simulink model "NoC_4x4x3"  (R2015a)
settings: Solver=ode45  StartTime=0.0  StopTime=10.0  RelTol=1e-3
undefined symbols (not defined in the file or in its folder): des, SELECT
undefined symbols (not defined in the file): MAX, MIN, T
libraries: simulink x48
(part 11 of 12)

== system NoC_4x4x3/LayerDown/Sitch3DXYZ/RouteXYZ/Attribute Function ==
  MATLAB Function : MATLAB Function  TreatAsAtomicUnit=on
  __DMLF__EDE2FCE__ : EntityDepartureFunctionCallGenerator  TimingFunctionCallF1=Before entity departure  IsInsideAFB=on
  __DMLF__GA__ : GetAttribute  AttributeName=DST_X|DST_Y|DST_Z|IME_X|IME_Y|IME_Z  AttributeMissing=Error|Error|Error|Error|Error|Error  AttributeDefaultValue=1|1|1|1|1|1  AttributeTreatAsVector=1|1|1|1|1|1  AttributeSendTiming=Before entity departure|Before entity departure|Before entity departure|Before entity departure|Before entity departure|Before entity departure  EvaluatedDefaultAttributeValue={ [];[];[];[];[];[]}  IsInsideAFB=on
      settings: OutputPortMap=o1,o2,o3,o4,o5,o6
  __DMLF__SA__ : SetAttribute  AttributeName=RT  AttributeFrom=Signal port  EvaluatedAttributeValue={ []}  IsInsideAFB=on
  IN : PMIOPort  Port=1  Side=Left
  OUT : PMIOPort  Port=2  Side=Right
  wires:
  __DMLF__EDE2FCE__/1 -> MATLAB Function/Trigger
  __DMLF__GA__/1 -> MATLAB Function/1(DST_X)
  __DMLF__GA__/2 -> MATLAB Function/2(DST_Y)
  __DMLF__GA__/3 -> MATLAB Function/3(DST_Z)
  __DMLF__GA__/4 -> MATLAB Function/4(IME_X)
  __DMLF__GA__/5 -> MATLAB Function/5(IME_Y)
  __DMLF__GA__/6 -> MATLAB Function/6(IME_Z)
  MATLAB Function/1(out_RT) -> __DMLF__SA__/1
  connections:
  __DMLF__SA__/RConn1 -- OUT/RConn1
  IN/RConn1 -- __DMLF__GA__/LConn1
  __DMLF__GA__/RConn1 -- __DMLF__EDE2FCE__/LConn1
  __DMLF__SA__/LConn1 -- __DMLF__EDE2FCE__/RConn1

== system NoC_4x4x3/LayerDown/Sitch3DXYZ1/RouteXYZ/Attribute Function ==
  MATLAB Function : MATLAB Function  TreatAsAtomicUnit=on
  __DMLF__EDE2FCE__ : EntityDepartureFunctionCallGenerator  TimingFunctionCallF1=Before entity departure  IsInsideAFB=on
  __DMLF__GA__ : GetAttribute  AttributeName=DST_X|DST_Y|DST_Z|IME_X|IME_Y|IME_Z  AttributeMissing=Error|Error|Error|Error|Error|Error  AttributeDefaultValue=1|1|1|1|1|1  AttributeTreatAsVector=1|1|1|1|1|1  AttributeSendTiming=Before entity departure|Before entity departure|Before entity departure|Before entity departure|Before entity departure|Before entity departure  EvaluatedDefaultAttributeValue={ [];[];[];[];[];[]}  IsInsideAFB=on
      settings: OutputPortMap=o1,o2,o3,o4,o5,o6
  __DMLF__SA__ : SetAttribute  AttributeName=RT  AttributeFrom=Signal port  EvaluatedAttributeValue={ []}  IsInsideAFB=on
  IN : PMIOPort  Port=1  Side=Left
  OUT : PMIOPort  Port=2  Side=Right
  wires:
  __DMLF__EDE2FCE__/1 -> MATLAB Function/Trigger
  __DMLF__GA__/1 -> MATLAB Function/1(DST_X)
  __DMLF__GA__/2 -> MATLAB Function/2(DST_Y)
  __DMLF__GA__/3 -> MATLAB Function/3(DST_Z)
  __DMLF__GA__/4 -> MATLAB Function/4(IME_X)
  __DMLF__GA__/5 -> MATLAB Function/5(IME_Y)
  __DMLF__GA__/6 -> MATLAB Function/6(IME_Z)
  MATLAB Function/1(out_RT) -> __DMLF__SA__/1
  connections:
  __DMLF__SA__/LConn1 -- __DMLF__EDE2FCE__/RConn1
  __DMLF__GA__/RConn1 -- __DMLF__EDE2FCE__/LConn1
  IN/RConn1 -- __DMLF__GA__/LConn1
  __DMLF__SA__/RConn1 -- OUT/RConn1

== system NoC_4x4x3/LayerDown/Sitch3DXYZ10/RouteXYZ/Attribute Function ==
  MATLAB Function : MATLAB Function  TreatAsAtomicUnit=on
  __DMLF__EDE2FCE__ : EntityDepartureFunctionCallGenerator  TimingFunctionCallF1=Before entity departure  IsInsideAFB=on
  __DMLF__GA__ : GetAttribute  AttributeName=DST_X|DST_Y|DST_Z|IME_X|IME_Y|IME_Z  AttributeMissing=Error|Error|Error|Error|Error|Error  AttributeDefaultValue=1|1|1|1|1|1  AttributeTreatAsVector=1|1|1|1|1|1  AttributeSendTiming=Before entity departure|Before entity departure|Before entity departure|Before entity departure|Before entity departure|Before entity departure  EvaluatedDefaultAttributeValue={ [];[];[];[];[];[]}  IsInsideAFB=on
      settings: OutputPortMap=o1,o2,o3,o4,o5,o6
  __DMLF__SA__ : SetAttribute  AttributeName=RT  AttributeFrom=Signal port  EvaluatedAttributeValue={ []}  IsInsideAFB=on
  IN : PMIOPort  Port=1  Side=Left
  OUT : PMIOPort  Port=2  Side=Right
  wires:
  __DMLF__EDE2FCE__/1 -> MATLAB Function/Trigger
  __DMLF__GA__/1 -> MATLAB Function/1(DST_X)
  __DMLF__GA__/2 -> MATLAB Function/2(DST_Y)
  __DMLF__GA__/3 -> MATLAB Function/3(DST_Z)
  __DMLF__GA__/4 -> MATLAB Function/4(IME_X)
  __DMLF__GA__/5 -> MATLAB Function/5(IME_Y)
  __DMLF__GA__/6 -> MATLAB Function/6(IME_Z)
  MATLAB Function/1(out_RT) -> __DMLF__SA__/1
  connections:
  __DMLF__SA__/RConn1 -- OUT/RConn1
  IN/RConn1 -- __DMLF__GA__/LConn1
  __DMLF__GA__/RConn1 -- __DMLF__EDE2FCE__/LConn1
  __DMLF__SA__/LConn1 -- __DMLF__EDE2FCE__/RConn1

== system NoC_4x4x3/LayerDown/Sitch3DXYZ11/RouteXYZ/Attribute Function ==
  MATLAB Function : MATLAB Function  TreatAsAtomicUnit=on
  __DMLF__EDE2FCE__ : EntityDepartureFunctionCallGenerator  TimingFunctionCallF1=Before entity departure  IsInsideAFB=on
  __DMLF__GA__ : GetAttribute  AttributeName=DST_X|DST_Y|DST_Z|IME_X|IME_Y|IME_Z  AttributeMissing=Error|Error|Error|Error|Error|Error  AttributeDefaultValue=1|1|1|1|1|1  AttributeTreatAsVector=1|1|1|1|1|1  AttributeSendTiming=Before entity departure|Before entity departure|Before entity departure|Before entity departure|Before entity departure|Before entity departure  EvaluatedDefaultAttributeValue={ [];[];[];[];[];[]}  IsInsideAFB=on
      settings: OutputPortMap=o1,o2,o3,o4,o5,o6
  __DMLF__SA__ : SetAttribute  AttributeName=RT  AttributeFrom=Signal port  EvaluatedAttributeValue={ []}  IsInsideAFB=on
  IN : PMIOPort  Port=1  Side=Left
  OUT : PMIOPort  Port=2  Side=Right
  wires:
  __DMLF__EDE2FCE__/1 -> MATLAB Function/Trigger
  __DMLF__GA__/1 -> MATLAB Function/1(DST_X)
  __DMLF__GA__/2 -> MATLAB Function/2(DST_Y)
  __DMLF__GA__/3 -> MATLAB Function/3(DST_Z)
  __DMLF__GA__/4 -> MATLAB Function/4(IME_X)
  __DMLF__GA__/5 -> MATLAB Function/5(IME_Y)
  __DMLF__GA__/6 -> MATLAB Function/6(IME_Z)
  MATLAB Function/1(out_RT) -> __DMLF__SA__/1
  connections:
  __DMLF__SA__/LConn1 -- __DMLF__EDE2FCE__/RConn1
  __DMLF__GA__/RConn1 -- __DMLF__EDE2FCE__/LConn1
  IN/RConn1 -- __DMLF__GA__/LConn1
  __DMLF__SA__/RConn1 -- OUT/RConn1

== system NoC_4x4x3/LayerDown/Sitch3DXYZ12/RouteXYZ/Attribute Function ==
  MATLAB Function : MATLAB Function  TreatAsAtomicUnit=on
  __DMLF__EDE2FCE__ : EntityDepartureFunctionCallGenerator  TimingFunctionCallF1=Before entity departure  IsInsideAFB=on
  __DMLF__GA__ : GetAttribute  AttributeName=DST_X|DST_Y|DST_Z|IME_X|IME_Y|IME_Z  AttributeMissing=Error|Error|Error|Error|Error|Error  AttributeDefaultValue=1|1|1|1|1|1  AttributeTreatAsVector=1|1|1|1|1|1  AttributeSendTiming=Before entity departure|Before entity departure|Before entity departure|Before entity departure|Before entity departure|Before entity departure  EvaluatedDefaultAttributeValue={ [];[];[];[];[];[]}  IsInsideAFB=on
      settings: OutputPortMap=o1,o2,o3,o4,o5,o6
  __DMLF__SA__ : SetAttribute  AttributeName=RT  AttributeFrom=Signal port  EvaluatedAttributeValue={ []}  IsInsideAFB=on
  IN : PMIOPort  Port=1  Side=Left
  OUT : PMIOPort  Port=2  Side=Right
  wires:
  __DMLF__EDE2FCE__/1 -> MATLAB Function/Trigger
  __DMLF__GA__/1 -> MATLAB Function/1(DST_X)
  __DMLF__GA__/2 -> MATLAB Function/2(DST_Y)
  __DMLF__GA__/3 -> MATLAB Function/3(DST_Z)
  __DMLF__GA__/4 -> MATLAB Function/4(IME_X)
  __DMLF__GA__/5 -> MATLAB Function/5(IME_Y)
  __DMLF__GA__/6 -> MATLAB Function/6(IME_Z)
  MATLAB Function/1(out_RT) -> __DMLF__SA__/1
  connections:
  __DMLF__SA__/LConn1 -- __DMLF__EDE2FCE__/RConn1
  __DMLF__GA__/RConn1 -- __DMLF__EDE2FCE__/LConn1
  IN/RConn1 -- __DMLF__GA__/LConn1
  __DMLF__SA__/RConn1 -- OUT/RConn1

== system NoC_4x4x3/LayerDown/Sitch3DXYZ13/RouteXYZ/Attribute Function ==
  MATLAB Function : MATLAB Function  TreatAsAtomicUnit=on
  __DMLF__EDE2FCE__ : EntityDepartureFunctionCallGenerator  TimingFunctionCallF1=Before entity departure  IsInsideAFB=on
  __DMLF__GA__ : GetAttribute  AttributeName=DST_X|DST_Y|DST_Z|IME_X|IME_Y|IME_Z  AttributeMissing=Error|Error|Error|Error|Error|Error  AttributeDefaultValue=1|1|1|1|1|1  AttributeTreatAsVector=1|1|1|1|1|1  AttributeSendTiming=Before entity departure|Before entity departure|Before entity departure|Before entity departure|Before entity departure|Before entity departure  EvaluatedDefaultAttributeValue={ [];[];[];[];[];[]}  IsInsideAFB=on
      settings: OutputPortMap=o1,o2,o3,o4,o5,o6
  __DMLF__SA__ : SetAttribute  AttributeName=RT  AttributeFrom=Signal port  EvaluatedAttributeValue={ []}  IsInsideAFB=on
  IN : PMIOPort  Port=1  Side=Left
  OUT : PMIOPort  Port=2  Side=Right
  wires:
  __DMLF__EDE2FCE__/1 -> MATLAB Function/Trigger
  __DMLF__GA__/1 -> MATLAB Function/1(DST_X)
  __DMLF__GA__/2 -> MATLAB Function/2(DST_Y)
  __DMLF__GA__/3 -> MATLAB Function/3(DST_Z)
  __DMLF__GA__/4 -> MATLAB Function/4(IME_X)
  __DMLF__GA__/5 -> MATLAB Function/5(IME_Y)
  __DMLF__GA__/6 -> MATLAB Function/6(IME_Z)
  MATLAB Function/1(out_RT) -> __DMLF__SA__/1
  connections:
  __DMLF__SA__/RConn1 -- OUT/RConn1
  IN/RConn1 -- __DMLF__GA__/LConn1
  __DMLF__GA__/RConn1 -- __DMLF__EDE2FCE__/LConn1
  __DMLF__SA__/LConn1 -- __DMLF__EDE2FCE__/RConn1

== system NoC_4x4x3/LayerDown/Sitch3DXYZ14/RouteXYZ/Attribute Function ==
  MATLAB Function : MATLAB Function  TreatAsAtomicUnit=on
  __DMLF__EDE2FCE__ : EntityDepartureFunctionCallGenerator  TimingFunctionCallF1=Before entity departure  IsInsideAFB=on
  __DMLF__GA__ : GetAttribute  AttributeName=DST_X|DST_Y|DST_Z|IME_X|IME_Y|IME_Z  AttributeMissing=Error|Error|Error|Error|Error|Error  AttributeDefaultValue=1|1|1|1|1|1  AttributeTreatAsVector=1|1|1|1|1|1  AttributeSendTiming=Before entity departure|Before entity departure|Before entity departure|Before entity departure|Before entity departure|Before entity departure  EvaluatedDefaultAttributeValue={ [];[];[];[];[];[]}  IsInsideAFB=on
      settings: OutputPortMap=o1,o2,o3,o4,o5,o6
  __DMLF__SA__ : SetAttribute  AttributeName=RT  AttributeFrom=Signal port  EvaluatedAttributeValue={ []}  IsInsideAFB=on
  IN : PMIOPort  Port=1  Side=Left
  OUT : PMIOPort  Port=2  Side=Right
  wires:
  __DMLF__EDE2FCE__/1 -> MATLAB Function/Trigger
  __DMLF__GA__/1 -> MATLAB Function/1(DST_X)
  __DMLF__GA__/2 -> MATLAB Function/2(DST_Y)
  __DMLF__GA__/3 -> MATLAB Function/3(DST_Z)
  __DMLF__GA__/4 -> MATLAB Function/4(IME_X)
  __DMLF__GA__/5 -> MATLAB Function/5(IME_Y)
  __DMLF__GA__/6 -> MATLAB Function/6(IME_Z)
  MATLAB Function/1(out_RT) -> __DMLF__SA__/1
  connections:
  __DMLF__SA__/LConn1 -- __DMLF__EDE2FCE__/RConn1
  __DMLF__GA__/RConn1 -- __DMLF__EDE2FCE__/LConn1
  IN/RConn1 -- __DMLF__GA__/LConn1
  __DMLF__SA__/RConn1 -- OUT/RConn1

== system NoC_4x4x3/LayerDown/Sitch3DXYZ15/RouteXYZ/Attribute Function ==
  MATLAB Function : MATLAB Function  TreatAsAtomicUnit=on
  __DMLF__EDE2FCE__ : EntityDepartureFunctionCallGenerator  TimingFunctionCallF1=Before entity departure  IsInsideAFB=on
  __DMLF__GA__ : GetAttribute  AttributeName=DST_X|DST_Y|DST_Z|IME_X|IME_Y|IME_Z  AttributeMissing=Error|Error|Error|Error|Error|Error  AttributeDefaultValue=1|1|1|1|1|1  AttributeTreatAsVector=1|1|1|1|1|1  AttributeSendTiming=Before entity departure|Before entity departure|Before entity departure|Before entity departure|Before entity departure|Before entity departure  EvaluatedDefaultAttributeValue={ [];[];[];[];[];[]}  IsInsideAFB=on
      settings: OutputPortMap=o1,o2,o3,o4,o5,o6
  __DMLF__SA__ : SetAttribute  AttributeName=RT  AttributeFrom=Signal port  EvaluatedAttributeValue={ []}  IsInsideAFB=on
  IN : PMIOPort  Port=1  Side=Left
  OUT : PMIOPort  Port=2  Side=Right
  wires:
  __DMLF__EDE2FCE__/1 -> MATLAB Function/Trigger
  __DMLF__GA__/1 -> MATLAB Function/1(DST_X)
  __DMLF__GA__/2 -> MATLAB Function/2(DST_Y)
  __DMLF__GA__/3 -> MATLAB Function/3(DST_Z)
  __DMLF__GA__/4 -> MATLAB Function/4(IME_X)
  __DMLF__GA__/5 -> MATLAB Function/5(IME_Y)
  __DMLF__GA__/6 -> MATLAB Function/6(IME_Z)
  MATLAB Function/1(out_RT) -> __DMLF__SA__/1
  connections:
  __DMLF__SA__/RConn1 -- OUT/RConn1
  IN/RConn1 -- __DMLF__GA__/LConn1
  __DMLF__GA__/RConn1 -- __DMLF__EDE2FCE__/LConn1
  __DMLF__SA__/LConn1 -- __DMLF__EDE2FCE__/RConn1

== system NoC_4x4x3/LayerDown/Sitch3DXYZ2/RouteXYZ/Attribute Function ==
  MATLAB Function : MATLAB Function  TreatAsAtomicUnit=on
  __DMLF__EDE2FCE__ : EntityDepartureFunctionCallGenerator  TimingFunctionCallF1=Before entity departure  IsInsideAFB=on
  __DMLF__GA__ : GetAttribute  AttributeName=DST_X|DST_Y|DST_Z|IME_X|IME_Y|IME_Z  AttributeMissing=Error|Error|Error|Error|Error|Error  AttributeDefaultValue=1|1|1|1|1|1  AttributeTreatAsVector=1|1|1|1|1|1  AttributeSendTiming=Before entity departure|Before entity departure|Before entity departure|Before entity departure|Before entity departure|Before entity departure  EvaluatedDefaultAttributeValue={ [];[];[];[];[];[]}  IsInsideAFB=on
      settings: OutputPortMap=o1,o2,o3,o4,o5,o6
  __DMLF__SA__ : SetAttribute  AttributeName=RT  AttributeFrom=Signal port  EvaluatedAttributeValue={ []}  IsInsideAFB=on
  IN : PMIOPort  Port=1  Side=Left
  OUT : PMIOPort  Port=2  Side=Right
  wires:
  __DMLF__EDE2FCE__/1 -> MATLAB Function/Trigger
  __DMLF__GA__/1 -> MATLAB Function/1(DST_X)
  __DMLF__GA__/2 -> MATLAB Function/2(DST_Y)
  __DMLF__GA__/3 -> MATLAB Function/3(DST_Z)
  __DMLF__GA__/4 -> MATLAB Function/4(IME_X)
  __DMLF__GA__/5 -> MATLAB Function/5(IME_Y)
  __DMLF__GA__/6 -> MATLAB Function/6(IME_Z)
  MATLAB Function/1(out_RT) -> __DMLF__SA__/1
  connections:
  __DMLF__SA__/RConn1 -- OUT/RConn1
  IN/RConn1 -- __DMLF__GA__/LConn1
  __DMLF__GA__/RConn1 -- __DMLF__EDE2FCE__/LConn1
  __DMLF__SA__/LConn1 -- __DMLF__EDE2FCE__/RConn1

== system NoC_4x4x3/LayerDown/Sitch3DXYZ3/RouteXYZ/Attribute Function ==
  MATLAB Function : MATLAB Function  TreatAsAtomicUnit=on
  __DMLF__EDE2FCE__ : EntityDepartureFunctionCallGenerator  TimingFunctionCallF1=Before entity departure  IsInsideAFB=on
  __DMLF__GA__ : GetAttribute  AttributeName=DST_X|DST_Y|DST_Z|IME_X|IME_Y|IME_Z  AttributeMissing=Error|Error|Error|Error|Error|Error  AttributeDefaultValue=1|1|1|1|1|1  AttributeTreatAsVector=1|1|1|1|1|1  AttributeSendTiming=Before entity departure|Before entity departure|Before entity departure|Before entity departure|Before entity departure|Before entity departure  EvaluatedDefaultAttributeValue={ [];[];[];[];[];[]}  IsInsideAFB=on
      settings: OutputPortMap=o1,o2,o3,o4,o5,o6
  __DMLF__SA__ : SetAttribute  AttributeName=RT  AttributeFrom=Signal port  EvaluatedAttributeValue={ []}  IsInsideAFB=on
  IN : PMIOPort  Port=1  Side=Left
  OUT : PMIOPort  Port=2  Side=Right
  wires:
  __DMLF__EDE2FCE__/1 -> MATLAB Function/Trigger
  __DMLF__GA__/1 -> MATLAB Function/1(DST_X)
  __DMLF__GA__/2 -> MATLAB Function/2(DST_Y)
  __DMLF__GA__/3 -> MATLAB Function/3(DST_Z)
  __DMLF__GA__/4 -> MATLAB Function/4(IME_X)
  __DMLF__GA__/5 -> MATLAB Function/5(IME_Y)
  __DMLF__GA__/6 -> MATLAB Function/6(IME_Z)
  MATLAB Function/1(out_RT) -> __DMLF__SA__/1
  connections:
  __DMLF__SA__/LConn1 -- __DMLF__EDE2FCE__/RConn1
  __DMLF__GA__/RConn1 -- __DMLF__EDE2FCE__/LConn1
  IN/RConn1 -- __DMLF__GA__/LConn1
  __DMLF__SA__/RConn1 -- OUT/RConn1

== system NoC_4x4x3/LayerDown/Sitch3DXYZ4/RouteXYZ/Attribute Function ==
  MATLAB Function : MATLAB Function  TreatAsAtomicUnit=on
  __DMLF__EDE2FCE__ : EntityDepartureFunctionCallGenerator  TimingFunctionCallF1=Before entity departure  IsInsideAFB=on
  __DMLF__GA__ : GetAttribute  AttributeName=DST_X|DST_Y|DST_Z|IME_X|IME_Y|IME_Z  AttributeMissing=Error|Error|Error|Error|Error|Error  AttributeDefaultValue=1|1|1|1|1|1  AttributeTreatAsVector=1|1|1|1|1|1  AttributeSendTiming=Before entity departure|Before entity departure|Before entity departure|Before entity departure|Before entity departure|Before entity departure  EvaluatedDefaultAttributeValue={ [];[];[];[];[];[]}  IsInsideAFB=on
      settings: OutputPortMap=o1,o2,o3,o4,o5,o6
  __DMLF__SA__ : SetAttribute  AttributeName=RT  AttributeFrom=Signal port  EvaluatedAttributeValue={ []}  IsInsideAFB=on
  IN : PMIOPort  Port=1  Side=Left
  OUT : PMIOPort  Port=2  Side=Right
  wires:
  __DMLF__EDE2FCE__/1 -> MATLAB Function/Trigger
  __DMLF__GA__/1 -> MATLAB Function/1(DST_X)
  __DMLF__GA__/2 -> MATLAB Function/2(DST_Y)
  __DMLF__GA__/3 -> MATLAB Function/3(DST_Z)
  __DMLF__GA__/4 -> MATLAB Function/4(IME_X)
  __DMLF__GA__/5 -> MATLAB Function/5(IME_Y)
  __DMLF__GA__/6 -> MATLAB Function/6(IME_Z)
  MATLAB Function/1(out_RT) -> __DMLF__SA__/1
  connections:
  __DMLF__SA__/LConn1 -- __DMLF__EDE2FCE__/RConn1
  __DMLF__GA__/RConn1 -- __DMLF__EDE2FCE__/LConn1
  IN/RConn1 -- __DMLF__GA__/LConn1
  __DMLF__SA__/RConn1 -- OUT/RConn1

== system NoC_4x4x3/LayerDown/Sitch3DXYZ5/RouteXYZ/Attribute Function ==
  MATLAB Function : MATLAB Function  TreatAsAtomicUnit=on
  __DMLF__EDE2FCE__ : EntityDepartureFunctionCallGenerator  TimingFunctionCallF1=Before entity departure  IsInsideAFB=on
  __DMLF__GA__ : GetAttribute  AttributeName=DST_X|DST_Y|DST_Z|IME_X|IME_Y|IME_Z  AttributeMissing=Error|Error|Error|Error|Error|Error  AttributeDefaultValue=1|1|1|1|1|1  AttributeTreatAsVector=1|1|1|1|1|1  AttributeSendTiming=Before entity departure|Before entity departure|Before entity departure|Before entity departure|Before entity departure|Before entity departure  EvaluatedDefaultAttributeValue={ [];[];[];[];[];[]}  IsInsideAFB=on
      settings: OutputPortMap=o1,o2,o3,o4,o5,o6
  __DMLF__SA__ : SetAttribute  AttributeName=RT  AttributeFrom=Signal port  EvaluatedAttributeValue={ []}  IsInsideAFB=on
  IN : PMIOPort  Port=1  Side=Left
  OUT : PMIOPort  Port=2  Side=Right
  wires:
  __DMLF__EDE2FCE__/1 -> MATLAB Function/Trigger
  __DMLF__GA__/1 -> MATLAB Function/1(DST_X)
  __DMLF__GA__/2 -> MATLAB Function/2(DST_Y)
  __DMLF__GA__/3 -> MATLAB Function/3(DST_Z)
  __DMLF__GA__/4 -> MATLAB Function/4(IME_X)
  __DMLF__GA__/5 -> MATLAB Function/5(IME_Y)
  __DMLF__GA__/6 -> MATLAB Function/6(IME_Z)
  MATLAB Function/1(out_RT) -> __DMLF__SA__/1
  connections:
  __DMLF__SA__/RConn1 -- OUT/RConn1
  IN/RConn1 -- __DMLF__GA__/LConn1
  __DMLF__GA__/RConn1 -- __DMLF__EDE2FCE__/LConn1
  __DMLF__SA__/LConn1 -- __DMLF__EDE2FCE__/RConn1

== system NoC_4x4x3/LayerDown/Sitch3DXYZ6/RouteXYZ/Attribute Function ==
  MATLAB Function : MATLAB Function  TreatAsAtomicUnit=on
  __DMLF__EDE2FCE__ : EntityDepartureFunctionCallGenerator  TimingFunctionCallF1=Before entity departure  IsInsideAFB=on
  __DMLF__GA__ : GetAttribute  AttributeName=DST_X|DST_Y|DST_Z|IME_X|IME_Y|IME_Z  AttributeMissing=Error|Error|Error|Error|Error|Error  AttributeDefaultValue=1|1|1|1|1|1  AttributeTreatAsVector=1|1|1|1|1|1  AttributeSendTiming=Before entity departure|Before entity departure|Before entity departure|Before entity departure|Before entity departure|Before entity departure  EvaluatedDefaultAttributeValue={ [];[];[];[];[];[]}  IsInsideAFB=on
      settings: OutputPortMap=o1,o2,o3,o4,o5,o6
  __DMLF__SA__ : SetAttribute  AttributeName=RT  AttributeFrom=Signal port  EvaluatedAttributeValue={ []}  IsInsideAFB=on
  IN : PMIOPort  Port=1  Side=Left
  OUT : PMIOPort  Port=2  Side=Right
  wires:
  __DMLF__EDE2FCE__/1 -> MATLAB Function/Trigger
  __DMLF__GA__/1 -> MATLAB Function/1(DST_X)
  __DMLF__GA__/2 -> MATLAB Function/2(DST_Y)
  __DMLF__GA__/3 -> MATLAB Function/3(DST_Z)
  __DMLF__GA__/4 -> MATLAB Function/4(IME_X)
  __DMLF__GA__/5 -> MATLAB Function/5(IME_Y)
  __DMLF__GA__/6 -> MATLAB Function/6(IME_Z)
  MATLAB Function/1(out_RT) -> __DMLF__SA__/1
  connections:
  __DMLF__SA__/LConn1 -- __DMLF__EDE2FCE__/RConn1
  __DMLF__GA__/RConn1 -- __DMLF__EDE2FCE__/LConn1
  IN/RConn1 -- __DMLF__GA__/LConn1
  __DMLF__SA__/RConn1 -- OUT/RConn1

== system NoC_4x4x3/LayerDown/Sitch3DXYZ7/RouteXYZ/Attribute Function ==
  MATLAB Function : MATLAB Function  TreatAsAtomicUnit=on
  __DMLF__EDE2FCE__ : EntityDepartureFunctionCallGenerator  TimingFunctionCallF1=Before entity departure  IsInsideAFB=on
  __DMLF__GA__ : GetAttribute  AttributeName=DST_X|DST_Y|DST_Z|IME_X|IME_Y|IME_Z  AttributeMissing=Error|Error|Error|Error|Error|Error  AttributeDefaultValue=1|1|1|1|1|1  AttributeTreatAsVector=1|1|1|1|1|1  AttributeSendTiming=Before entity departure|Before entity departure|Before entity departure|Before entity departure|Before entity departure|Before entity departure  EvaluatedDefaultAttributeValue={ [];[];[];[];[];[]}  IsInsideAFB=on
      settings: OutputPortMap=o1,o2,o3,o4,o5,o6
  __DMLF__SA__ : SetAttribute  AttributeName=RT  AttributeFrom=Signal port  EvaluatedAttributeValue={ []}  IsInsideAFB=on
  IN : PMIOPort  Port=1  Side=Left
  OUT : PMIOPort  Port=2  Side=Right
  wires:
  __DMLF__EDE2FCE__/1 -> MATLAB Function/Trigger
  __DMLF__GA__/1 -> MATLAB Function/1(DST_X)
  __DMLF__GA__/2 -> MATLAB Function/2(DST_Y)
  __DMLF__GA__/3 -> MATLAB Function/3(DST_Z)
  __DMLF__GA__/4 -> MATLAB Function/4(IME_X)
  __DMLF__GA__/5 -> MATLAB Function/5(IME_Y)
  __DMLF__GA__/6 -> MATLAB Function/6(IME_Z)
  MATLAB Function/1(out_RT) -> __DMLF__SA__/1
  connections:
  __DMLF__SA__/RConn1 -- OUT/RConn1
  IN/RConn1 -- __DMLF__GA__/LConn1
  __DMLF__GA__/RConn1 -- __DMLF__EDE2FCE__/LConn1
  __DMLF__SA__/LConn1 -- __DMLF__EDE2FCE__/RConn1

== system NoC_4x4x3/LayerDown/Sitch3DXYZ8/RouteXYZ/Attribute Function ==
  MATLAB Function : MATLAB Function  TreatAsAtomicUnit=on
  __DMLF__EDE2FCE__ : EntityDepartureFunctionCallGenerator  TimingFunctionCallF1=Before entity departure  IsInsideAFB=on
  __DMLF__GA__ : GetAttribute  AttributeName=DST_X|DST_Y|DST_Z|IME_X|IME_Y|IME_Z  AttributeMissing=Error|Error|Error|Error|Error|Error  AttributeDefaultValue=1|1|1|1|1|1  AttributeTreatAsVector=1|1|1|1|1|1  AttributeSendTiming=Before entity departure|Before entity departure|Before entity departure|Before entity departure|Before entity departure|Before entity departure  EvaluatedDefaultAttributeValue={ [];[];[];[];[];[]}  IsInsideAFB=on
      settings: OutputPortMap=o1,o2,o3,o4,o5,o6
  __DMLF__SA__ : SetAttribute  AttributeName=RT  AttributeFrom=Signal port  EvaluatedAttributeValue={ []}  IsInsideAFB=on
  IN : PMIOPort  Port=1  Side=Left
  OUT : PMIOPort  Port=2  Side=Right
  wires:
  __DMLF__EDE2FCE__/1 -> MATLAB Function/Trigger
  __DMLF__GA__/1 -> MATLAB Function/1(DST_X)
  __DMLF__GA__/2 -> MATLAB Function/2(DST_Y)
  __DMLF__GA__/3 -> MATLAB Function/3(DST_Z)
  __DMLF__GA__/4 -> MATLAB Function/4(IME_X)
  __DMLF__GA__/5 -> MATLAB Function/5(IME_Y)
  __DMLF__GA__/6 -> MATLAB Function/6(IME_Z)
  MATLAB Function/1(out_RT) -> __DMLF__SA__/1
  connections:
  __DMLF__SA__/RConn1 -- OUT/RConn1
  IN/RConn1 -- __DMLF__GA__/LConn1
  __DMLF__GA__/RConn1 -- __DMLF__EDE2FCE__/LConn1
  __DMLF__SA__/LConn1 -- __DMLF__EDE2FCE__/RConn1

== system NoC_4x4x3/LayerDown/Sitch3DXYZ9/RouteXYZ/Attribute Function ==
  MATLAB Function : MATLAB Function  TreatAsAtomicUnit=on
  __DMLF__EDE2FCE__ : EntityDepartureFunctionCallGenerator  TimingFunctionCallF1=Before entity departure  IsInsideAFB=on
  __DMLF__GA__ : GetAttribute  AttributeName=DST_X|DST_Y|DST_Z|IME_X|IME_Y|IME_Z  AttributeMissing=Error|Error|Error|Error|Error|Error  AttributeDefaultValue=1|1|1|1|1|1  AttributeTreatAsVector=1|1|1|1|1|1  AttributeSendTiming=Before entity departure|Before entity departure|Before entity departure|Before entity departure|Before entity departure|Before entity departure  EvaluatedDefaultAttributeValue={ [];[];[];[];[];[]}  IsInsideAFB=on
      settings: OutputPortMap=o1,o2,o3,o4,o5,o6
  __DMLF__SA__ : SetAttribute  AttributeName=RT  AttributeFrom=Signal port  EvaluatedAttributeValue={ []}  IsInsideAFB=on
  IN : PMIOPort  Port=1  Side=Left
  OUT : PMIOPort  Port=2  Side=Right
  wires:
  __DMLF__EDE2FCE__/1 -> MATLAB Function/Trigger
  __DMLF__GA__/1 -> MATLAB Function/1(DST_X)
  __DMLF__GA__/2 -> MATLAB Function/2(DST_Y)
  __DMLF__GA__/3 -> MATLAB Function/3(DST_Z)
  __DMLF__GA__/4 -> MATLAB Function/4(IME_X)
  __DMLF__GA__/5 -> MATLAB Function/5(IME_Y)
  __DMLF__GA__/6 -> MATLAB Function/6(IME_Z)
  MATLAB Function/1(out_RT) -> __DMLF__SA__/1
  connections:
  __DMLF__SA__/LConn1 -- __DMLF__EDE2FCE__/RConn1
  __DMLF__GA__/RConn1 -- __DMLF__EDE2FCE__/LConn1
  IN/RConn1 -- __DMLF__GA__/LConn1
  __DMLF__SA__/RConn1 -- OUT/RConn1

== system NoC_4x4x3/LayerUp/Sitch3DXYZ/RouteXYZ/Attribute Function ==
  MATLAB Function : MATLAB Function  TreatAsAtomicUnit=on
  __DMLF__EDE2FCE__ : EntityDepartureFunctionCallGenerator  TimingFunctionCallF1=Before entity departure  IsInsideAFB=on
  __DMLF__GA__ : GetAttribute  AttributeName=DST_X|DST_Y|DST_Z|IME_X|IME_Y|IME_Z  AttributeMissing=Error|Error|Error|Error|Error|Error  AttributeDefaultValue=1|1|1|1|1|1  AttributeTreatAsVector=1|1|1|1|1|1  AttributeSendTiming=Before entity departure|Before entity departure|Before entity departure|Before entity departure|Before entity departure|Before entity departure  EvaluatedDefaultAttributeValue={ [];[];[];[];[];[]}  IsInsideAFB=on
      settings: OutputPortMap=o1,o2,o3,o4,o5,o6
  __DMLF__SA__ : SetAttribute  AttributeName=RT  AttributeFrom=Signal port  EvaluatedAttributeValue={ []}  IsInsideAFB=on
  IN : PMIOPort  Port=1  Side=Left
  OUT : PMIOPort  Port=2  Side=Right
  wires:
  __DMLF__EDE2FCE__/1 -> MATLAB Function/Trigger
  __DMLF__GA__/1 -> MATLAB Function/1(DST_X)
  __DMLF__GA__/2 -> MATLAB Function/2(DST_Y)
  __DMLF__GA__/3 -> MATLAB Function/3(DST_Z)
  __DMLF__GA__/4 -> MATLAB Function/4(IME_X)
  __DMLF__GA__/5 -> MATLAB Function/5(IME_Y)
  __DMLF__GA__/6 -> MATLAB Function/6(IME_Z)
  MATLAB Function/1(out_RT) -> __DMLF__SA__/1
  connections:
  __DMLF__SA__/RConn1 -- OUT/RConn1
  IN/RConn1 -- __DMLF__GA__/LConn1
  __DMLF__GA__/RConn1 -- __DMLF__EDE2FCE__/LConn1
  __DMLF__SA__/LConn1 -- __DMLF__EDE2FCE__/RConn1

== system NoC_4x4x3/LayerUp/Sitch3DXYZ1/RouteXYZ/Attribute Function ==
  MATLAB Function : MATLAB Function  TreatAsAtomicUnit=on
  __DMLF__EDE2FCE__ : EntityDepartureFunctionCallGenerator  TimingFunctionCallF1=Before entity departure  IsInsideAFB=on
  __DMLF__GA__ : GetAttribute  AttributeName=DST_X|DST_Y|DST_Z|IME_X|IME_Y|IME_Z  AttributeMissing=Error|Error|Error|Error|Error|Error  AttributeDefaultValue=1|1|1|1|1|1  AttributeTreatAsVector=1|1|1|1|1|1  AttributeSendTiming=Before entity departure|Before entity departure|Before entity departure|Before entity departure|Before entity departure|Before entity departure  EvaluatedDefaultAttributeValue={ [];[];[];[];[];[]}  IsInsideAFB=on
      settings: OutputPortMap=o1,o2,o3,o4,o5,o6
  __DMLF__SA__ : SetAttribute  AttributeName=RT  AttributeFrom=Signal port  EvaluatedAttributeValue={ []}  IsInsideAFB=on
  IN : PMIOPort  Port=1  Side=Left
  OUT : PMIOPort  Port=2  Side=Right
  wires:
  __DMLF__EDE2FCE__/1 -> MATLAB Function/Trigger
  __DMLF__GA__/1 -> MATLAB Function/1(DST_X)
  __DMLF__GA__/2 -> MATLAB Function/2(DST_Y)
  __DMLF__GA__/3 -> MATLAB Function/3(DST_Z)
  __DMLF__GA__/4 -> MATLAB Function/4(IME_X)
  __DMLF__GA__/5 -> MATLAB Function/5(IME_Y)
  __DMLF__GA__/6 -> MATLAB Function/6(IME_Z)
  MATLAB Function/1(out_RT) -> __DMLF__SA__/1
  connections:
  __DMLF__SA__/LConn1 -- __DMLF__EDE2FCE__/RConn1
  __DMLF__GA__/RConn1 -- __DMLF__EDE2FCE__/LConn1
  IN/RConn1 -- __DMLF__GA__/LConn1
  __DMLF__SA__/RConn1 -- OUT/RConn1

== system NoC_4x4x3/LayerUp/Sitch3DXYZ10/RouteXYZ/Attribute Function ==
  MATLAB Function : MATLAB Function  TreatAsAtomicUnit=on
  __DMLF__EDE2FCE__ : EntityDepartureFunctionCallGenerator  TimingFunctionCallF1=Before entity departure  IsInsideAFB=on
  __DMLF__GA__ : GetAttribute  AttributeName=DST_X|DST_Y|DST_Z|IME_X|IME_Y|IME_Z  AttributeMissing=Error|Error|Error|Error|Error|Error  AttributeDefaultValue=1|1|1|1|1|1  AttributeTreatAsVector=1|1|1|1|1|1  AttributeSendTiming=Before entity departure|Before entity departure|Before entity departure|Before entity departure|Before entity departure|Before entity departure  EvaluatedDefaultAttributeValue={ [];[];[];[];[];[]}  IsInsideAFB=on
      settings: OutputPortMap=o1,o2,o3,o4,o5,o6
  __DMLF__SA__ : SetAttribute  AttributeName=RT  AttributeFrom=Signal port  EvaluatedAttributeValue={ []}  IsInsideAFB=on
  IN : PMIOPort  Port=1  Side=Left
  OUT : PMIOPort  Port=2  Side=Right
  wires:
  __DMLF__EDE2FCE__/1 -> MATLAB Function/Trigger
  __DMLF__GA__/1 -> MATLAB Function/1(DST_X)
  __DMLF__GA__/2 -> MATLAB Function/2(DST_Y)
  __DMLF__GA__/3 -> MATLAB Function/3(DST_Z)
  __DMLF__GA__/4 -> MATLAB Function/4(IME_X)
  __DMLF__GA__/5 -> MATLAB Function/5(IME_Y)
  __DMLF__GA__/6 -> MATLAB Function/6(IME_Z)
  MATLAB Function/1(out_RT) -> __DMLF__SA__/1
  connections:
  __DMLF__SA__/RConn1 -- OUT/RConn1
  IN/RConn1 -- __DMLF__GA__/LConn1
  __DMLF__GA__/RConn1 -- __DMLF__EDE2FCE__/LConn1
  __DMLF__SA__/LConn1 -- __DMLF__EDE2FCE__/RConn1

== system NoC_4x4x3/LayerUp/Sitch3DXYZ11/RouteXYZ/Attribute Function ==
  MATLAB Function : MATLAB Function  TreatAsAtomicUnit=on
  __DMLF__EDE2FCE__ : EntityDepartureFunctionCallGenerator  TimingFunctionCallF1=Before entity departure  IsInsideAFB=on
  __DMLF__GA__ : GetAttribute  AttributeName=DST_X|DST_Y|DST_Z|IME_X|IME_Y|IME_Z  AttributeMissing=Error|Error|Error|Error|Error|Error  AttributeDefaultValue=1|1|1|1|1|1  AttributeTreatAsVector=1|1|1|1|1|1  AttributeSendTiming=Before entity departure|Before entity departure|Before entity departure|Before entity departure|Before entity departure|Before entity departure  EvaluatedDefaultAttributeValue={ [];[];[];[];[];[]}  IsInsideAFB=on
      settings: OutputPortMap=o1,o2,o3,o4,o5,o6
  __DMLF__SA__ : SetAttribute  AttributeName=RT  AttributeFrom=Signal port  EvaluatedAttributeValue={ []}  IsInsideAFB=on
  IN : PMIOPort  Port=1  Side=Left
  OUT : PMIOPort  Port=2  Side=Right
  wires:
  __DMLF__EDE2FCE__/1 -> MATLAB Function/Trigger
  __DMLF__GA__/1 -> MATLAB Function/1(DST_X)
  __DMLF__GA__/2 -> MATLAB Function/2(DST_Y)
  __DMLF__GA__/3 -> MATLAB Function/3(DST_Z)
  __DMLF__GA__/4 -> MATLAB Function/4(IME_X)
  __DMLF__GA__/5 -> MATLAB Function/5(IME_Y)
  __DMLF__GA__/6 -> MATLAB Function/6(IME_Z)
  MATLAB Function/1(out_RT) -> __DMLF__SA__/1
  connections:
  __DMLF__SA__/LConn1 -- __DMLF__EDE2FCE__/RConn1
  __DMLF__GA__/RConn1 -- __DMLF__EDE2FCE__/LConn1
  IN/RConn1 -- __DMLF__GA__/LConn1
  __DMLF__SA__/RConn1 -- OUT/RConn1

== system NoC_4x4x3/LayerUp/Sitch3DXYZ12/RouteXYZ/Attribute Function ==
  MATLAB Function : MATLAB Function  TreatAsAtomicUnit=on
  __DMLF__EDE2FCE__ : EntityDepartureFunctionCallGenerator  TimingFunctionCallF1=Before entity departure  IsInsideAFB=on
  __DMLF__GA__ : GetAttribute  AttributeName=DST_X|DST_Y|DST_Z|IME_X|IME_Y|IME_Z  AttributeMissing=Error|Error|Error|Error|Error|Error  AttributeDefaultValue=1|1|1|1|1|1  AttributeTreatAsVector=1|1|1|1|1|1  AttributeSendTiming=Before entity departure|Before entity departure|Before entity departure|Before entity departure|Before entity departure|Before entity departure  EvaluatedDefaultAttributeValue={ [];[];[];[];[];[]}  IsInsideAFB=on
      settings: OutputPortMap=o1,o2,o3,o4,o5,o6
  __DMLF__SA__ : SetAttribute  AttributeName=RT  AttributeFrom=Signal port  EvaluatedAttributeValue={ []}  IsInsideAFB=on
  IN : PMIOPort  Port=1  Side=Left
  OUT : PMIOPort  Port=2  Side=Right
  wires:
  __DMLF__EDE2FCE__/1 -> MATLAB Function/Trigger
  __DMLF__GA__/1 -> MATLAB Function/1(DST_X)
  __DMLF__GA__/2 -> MATLAB Function/2(DST_Y)
  __DMLF__GA__/3 -> MATLAB Function/3(DST_Z)
  __DMLF__GA__/4 -> MATLAB Function/4(IME_X)
  __DMLF__GA__/5 -> MATLAB Function/5(IME_Y)
  __DMLF__GA__/6 -> MATLAB Function/6(IME_Z)
  MATLAB Function/1(out_RT) -> __DMLF__SA__/1
  connections:
  __DMLF__SA__/LConn1 -- __DMLF__EDE2FCE__/RConn1
  __DMLF__GA__/RConn1 -- __DMLF__EDE2FCE__/LConn1
  IN/RConn1 -- __DMLF__GA__/LConn1
  __DMLF__SA__/RConn1 -- OUT/RConn1

== system NoC_4x4x3/LayerUp/Sitch3DXYZ13/RouteXYZ/Attribute Function ==
  MATLAB Function : MATLAB Function  TreatAsAtomicUnit=on
  __DMLF__EDE2FCE__ : EntityDepartureFunctionCallGenerator  TimingFunctionCallF1=Before entity departure  IsInsideAFB=on
  __DMLF__GA__ : GetAttribute  AttributeName=DST_X|DST_Y|DST_Z|IME_X|IME_Y|IME_Z  AttributeMissing=Error|Error|Error|Error|Error|Error  AttributeDefaultValue=1|1|1|1|1|1  AttributeTreatAsVector=1|1|1|1|1|1  AttributeSendTiming=Before entity departure|Before entity departure|Before entity departure|Before entity departure|Before entity departure|Before entity departure  EvaluatedDefaultAttributeValue={ [];[];[];[];[];[]}  IsInsideAFB=on
      settings: OutputPortMap=o1,o2,o3,o4,o5,o6
  __DMLF__SA__ : SetAttribute  AttributeName=RT  AttributeFrom=Signal port  EvaluatedAttributeValue={ []}  IsInsideAFB=on
  IN : PMIOPort  Port=1  Side=Left
  OUT : PMIOPort  Port=2  Side=Right
  wires:
  __DMLF__EDE2FCE__/1 -> MATLAB Function/Trigger
  __DMLF__GA__/1 -> MATLAB Function/1(DST_X)
  __DMLF__GA__/2 -> MATLAB Function/2(DST_Y)
  __DMLF__GA__/3 -> MATLAB Function/3(DST_Z)
  __DMLF__GA__/4 -> MATLAB Function/4(IME_X)
  __DMLF__GA__/5 -> MATLAB Function/5(IME_Y)
  __DMLF__GA__/6 -> MATLAB Function/6(IME_Z)
  MATLAB Function/1(out_RT) -> __DMLF__SA__/1
  connections:
  __DMLF__SA__/RConn1 -- OUT/RConn1
  IN/RConn1 -- __DMLF__GA__/LConn1
  __DMLF__GA__/RConn1 -- __DMLF__EDE2FCE__/LConn1
  __DMLF__SA__/LConn1 -- __DMLF__EDE2FCE__/RConn1

== system NoC_4x4x3/LayerUp/Sitch3DXYZ14/RouteXYZ/Attribute Function ==
  MATLAB Function : MATLAB Function  TreatAsAtomicUnit=on
  __DMLF__EDE2FCE__ : EntityDepartureFunctionCallGenerator  TimingFunctionCallF1=Before entity departure  IsInsideAFB=on
  __DMLF__GA__ : GetAttribute  AttributeName=DST_X|DST_Y|DST_Z|IME_X|IME_Y|IME_Z  AttributeMissing=Error|Error|Error|Error|Error|Error  AttributeDefaultValue=1|1|1|1|1|1  AttributeTreatAsVector=1|1|1|1|1|1  AttributeSendTiming=Before entity departure|Before entity departure|Before entity departure|Before entity departure|Before entity departure|Before entity departure  EvaluatedDefaultAttributeValue={ [];[];[];[];[];[]}  IsInsideAFB=on
      settings: OutputPortMap=o1,o2,o3,o4,o5,o6
  __DMLF__SA__ : SetAttribute  AttributeName=RT  AttributeFrom=Signal port  EvaluatedAttributeValue={ []}  IsInsideAFB=on
  IN : PMIOPort  Port=1  Side=Left
  OUT : PMIOPort  Port=2  Side=Right
  wires:
  __DMLF__EDE2FCE__/1 -> MATLAB Function/Trigger
  __DMLF__GA__/1 -> MATLAB Function/1(DST_X)
  __DMLF__GA__/2 -> MATLAB Function/2(DST_Y)
  __DMLF__GA__/3 -> MATLAB Function/3(DST_Z)
  __DMLF__GA__/4 -> MATLAB Function/4(IME_X)
  __DMLF__GA__/5 -> MATLAB Function/5(IME_Y)
  __DMLF__GA__/6 -> MATLAB Function/6(IME_Z)
  MATLAB Function/1(out_RT) -> __DMLF__SA__/1
  connections:
  __DMLF__SA__/LConn1 -- __DMLF__EDE2FCE__/RConn1
  __DMLF__GA__/RConn1 -- __DMLF__EDE2FCE__/LConn1
  IN/RConn1 -- __DMLF__GA__/LConn1
  __DMLF__SA__/RConn1 -- OUT/RConn1

== system NoC_4x4x3/LayerUp/Sitch3DXYZ15/RouteXYZ/Attribute Function ==
  MATLAB Function : MATLAB Function  TreatAsAtomicUnit=on
  __DMLF__EDE2FCE__ : EntityDepartureFunctionCallGenerator  TimingFunctionCallF1=Before entity departure  IsInsideAFB=on
  __DMLF__GA__ : GetAttribute  AttributeName=DST_X|DST_Y|DST_Z|IME_X|IME_Y|IME_Z  AttributeMissing=Error|Error|Error|Error|Error|Error  AttributeDefaultValue=1|1|1|1|1|1  AttributeTreatAsVector=1|1|1|1|1|1  AttributeSendTiming=Before entity departure|Before entity departure|Before entity departure|Before entity departure|Before entity departure|Before entity departure  EvaluatedDefaultAttributeValue={ [];[];[];[];[];[]}  IsInsideAFB=on
      settings: OutputPortMap=o1,o2,o3,o4,o5,o6
  __DMLF__SA__ : SetAttribute  AttributeName=RT  AttributeFrom=Signal port  EvaluatedAttributeValue={ []}  IsInsideAFB=on
  IN : PMIOPort  Port=1  Side=Left
  OUT : PMIOPort  Port=2  Side=Right
  wires:
  __DMLF__EDE2FCE__/1 -> MATLAB Function/Trigger
  __DMLF__GA__/1 -> MATLAB Function/1(DST_X)
  __DMLF__GA__/2 -> MATLAB Function/2(DST_Y)
  __DMLF__GA__/3 -> MATLAB Function/3(DST_Z)
  __DMLF__GA__/4 -> MATLAB Function/4(IME_X)
  __DMLF__GA__/5 -> MATLAB Function/5(IME_Y)
  __DMLF__GA__/6 -> MATLAB Function/6(IME_Z)
  MATLAB Function/1(out_RT) -> __DMLF__SA__/1
  connections:
  __DMLF__SA__/RConn1 -- OUT/RConn1
  IN/RConn1 -- __DMLF__GA__/LConn1
  __DMLF__GA__/RConn1 -- __DMLF__EDE2FCE__/LConn1
  __DMLF__SA__/LConn1 -- __DMLF__EDE2FCE__/RConn1

== system NoC_4x4x3/LayerUp/Sitch3DXYZ2/RouteXYZ/Attribute Function ==
  MATLAB Function : MATLAB Function  TreatAsAtomicUnit=on
  __DMLF__EDE2FCE__ : EntityDepartureFunctionCallGenerator  TimingFunctionCallF1=Before entity departure  IsInsideAFB=on
  __DMLF__GA__ : GetAttribute  AttributeName=DST_X|DST_Y|DST_Z|IME_X|IME_Y|IME_Z  AttributeMissing=Error|Error|Error|Error|Error|Error  AttributeDefaultValue=1|1|1|1|1|1  AttributeTreatAsVector=1|1|1|1|1|1  AttributeSendTiming=Before entity departure|Before entity departure|Before entity departure|Before entity departure|Before entity departure|Before entity departure  EvaluatedDefaultAttributeValue={ [];[];[];[];[];[]}  IsInsideAFB=on
      settings: OutputPortMap=o1,o2,o3,o4,o5,o6
  __DMLF__SA__ : SetAttribute  AttributeName=RT  AttributeFrom=Signal port  EvaluatedAttributeValue={ []}  IsInsideAFB=on
  IN : PMIOPort  Port=1  Side=Left
  OUT : PMIOPort  Port=2  Side=Right
  wires:
  __DMLF__EDE2FCE__/1 -> MATLAB Function/Trigger
  __DMLF__GA__/1 -> MATLAB Function/1(DST_X)
  __DMLF__GA__/2 -> MATLAB Function/2(DST_Y)
  __DMLF__GA__/3 -> MATLAB Function/3(DST_Z)
  __DMLF__GA__/4 -> MATLAB Function/4(IME_X)
  __DMLF__GA__/5 -> MATLAB Function/5(IME_Y)
  __DMLF__GA__/6 -> MATLAB Function/6(IME_Z)
  MATLAB Function/1(out_RT) -> __DMLF__SA__/1
  connections:
  __DMLF__SA__/RConn1 -- OUT/RConn1
  IN/RConn1 -- __DMLF__GA__/LConn1
  __DMLF__GA__/RConn1 -- __DMLF__EDE2FCE__/LConn1
  __DMLF__SA__/LConn1 -- __DMLF__EDE2FCE__/RConn1

== system NoC_4x4x3/LayerUp/Sitch3DXYZ3/RouteXYZ/Attribute Function ==
  MATLAB Function : MATLAB Function  TreatAsAtomicUnit=on
  __DMLF__EDE2FCE__ : EntityDepartureFunctionCallGenerator  TimingFunctionCallF1=Before entity departure  IsInsideAFB=on
  __DMLF__GA__ : GetAttribute  AttributeName=DST_X|DST_Y|DST_Z|IME_X|IME_Y|IME_Z  AttributeMissing=Error|Error|Error|Error|Error|Error  AttributeDefaultValue=1|1|1|1|1|1  AttributeTreatAsVector=1|1|1|1|1|1  AttributeSendTiming=Before entity departure|Before entity departure|Before entity departure|Before entity departure|Before entity departure|Before entity departure  EvaluatedDefaultAttributeValue={ [];[];[];[];[];[]}  IsInsideAFB=on
      settings: OutputPortMap=o1,o2,o3,o4,o5,o6
  __DMLF__SA__ : SetAttribute  AttributeName=RT  AttributeFrom=Signal port  EvaluatedAttributeValue={ []}  IsInsideAFB=on
  IN : PMIOPort  Port=1  Side=Left
  OUT : PMIOPort  Port=2  Side=Right
  wires:
  __DMLF__EDE2FCE__/1 -> MATLAB Function/Trigger
  __DMLF__GA__/1 -> MATLAB Function/1(DST_X)
  __DMLF__GA__/2 -> MATLAB Function/2(DST_Y)
  __DMLF__GA__/3 -> MATLAB Function/3(DST_Z)
  __DMLF__GA__/4 -> MATLAB Function/4(IME_X)
  __DMLF__GA__/5 -> MATLAB Function/5(IME_Y)
  __DMLF__GA__/6 -> MATLAB Function/6(IME_Z)
  MATLAB Function/1(out_RT) -> __DMLF__SA__/1
  connections:
  __DMLF__SA__/LConn1 -- __DMLF__EDE2FCE__/RConn1
  __DMLF__GA__/RConn1 -- __DMLF__EDE2FCE__/LConn1
  IN/RConn1 -- __DMLF__GA__/LConn1
  __DMLF__SA__/RConn1 -- OUT/RConn1

== system NoC_4x4x3/LayerUp/Sitch3DXYZ4/RouteXYZ/Attribute Function ==
  MATLAB Function : MATLAB Function  TreatAsAtomicUnit=on
  __DMLF__EDE2FCE__ : EntityDepartureFunctionCallGenerator  TimingFunctionCallF1=Before entity departure  IsInsideAFB=on
  __DMLF__GA__ : GetAttribute  AttributeName=DST_X|DST_Y|DST_Z|IME_X|IME_Y|IME_Z  AttributeMissing=Error|Error|Error|Error|Error|Error  AttributeDefaultValue=1|1|1|1|1|1  AttributeTreatAsVector=1|1|1|1|1|1  AttributeSendTiming=Before entity departure|Before entity departure|Before entity departure|Before entity departure|Before entity departure|Before entity departure  EvaluatedDefaultAttributeValue={ [];[];[];[];[];[]}  IsInsideAFB=on
      settings: OutputPortMap=o1,o2,o3,o4,o5,o6
  __DMLF__SA__ : SetAttribute  AttributeName=RT  AttributeFrom=Signal port  EvaluatedAttributeValue={ []}  IsInsideAFB=on
  IN : PMIOPort  Port=1  Side=Left
  OUT : PMIOPort  Port=2  Side=Right
  wires:
  __DMLF__EDE2FCE__/1 -> MATLAB Function/Trigger
  __DMLF__GA__/1 -> MATLAB Function/1(DST_X)
  __DMLF__GA__/2 -> MATLAB Function/2(DST_Y)
  __DMLF__GA__/3 -> MATLAB Function/3(DST_Z)
  __DMLF__GA__/4 -> MATLAB Function/4(IME_X)
  __DMLF__GA__/5 -> MATLAB Function/5(IME_Y)
  __DMLF__GA__/6 -> MATLAB Function/6(IME_Z)
  MATLAB Function/1(out_RT) -> __DMLF__SA__/1
  connections:
  __DMLF__SA__/LConn1 -- __DMLF__EDE2FCE__/RConn1
  __DMLF__GA__/RConn1 -- __DMLF__EDE2FCE__/LConn1
  IN/RConn1 -- __DMLF__GA__/LConn1
  __DMLF__SA__/RConn1 -- OUT/RConn1

== system NoC_4x4x3/LayerUp/Sitch3DXYZ5/RouteXYZ/Attribute Function ==
  MATLAB Function : MATLAB Function  TreatAsAtomicUnit=on
  __DMLF__EDE2FCE__ : EntityDepartureFunctionCallGenerator  TimingFunctionCallF1=Before entity departure  IsInsideAFB=on
  __DMLF__GA__ : GetAttribute  AttributeName=DST_X|DST_Y|DST_Z|IME_X|IME_Y|IME_Z  AttributeMissing=Error|Error|Error|Error|Error|Error  AttributeDefaultValue=1|1|1|1|1|1  AttributeTreatAsVector=1|1|1|1|1|1  AttributeSendTiming=Before entity departure|Before entity departure|Before entity departure|Before entity departure|Before entity departure|Before entity departure  EvaluatedDefaultAttributeValue={ [];[];[];[];[];[]}  IsInsideAFB=on
      settings: OutputPortMap=o1,o2,o3,o4,o5,o6
  __DMLF__SA__ : SetAttribute  AttributeName=RT  AttributeFrom=Signal port  EvaluatedAttributeValue={ []}  IsInsideAFB=on
  IN : PMIOPort  Port=1  Side=Left
  OUT : PMIOPort  Port=2  Side=Right
  wires:
  __DMLF__EDE2FCE__/1 -> MATLAB Function/Trigger
  __DMLF__GA__/1 -> MATLAB Function/1(DST_X)
  __DMLF__GA__/2 -> MATLAB Function/2(DST_Y)
  __DMLF__GA__/3 -> MATLAB Function/3(DST_Z)
  __DMLF__GA__/4 -> MATLAB Function/4(IME_X)
  __DMLF__GA__/5 -> MATLAB Function/5(IME_Y)
  __DMLF__GA__/6 -> MATLAB Function/6(IME_Z)
  MATLAB Function/1(out_RT) -> __DMLF__SA__/1
  connections:
  __DMLF__SA__/RConn1 -- OUT/RConn1
  IN/RConn1 -- __DMLF__GA__/LConn1
  __DMLF__GA__/RConn1 -- __DMLF__EDE2FCE__/LConn1
  __DMLF__SA__/LConn1 -- __DMLF__EDE2FCE__/RConn1

== system NoC_4x4x3/LayerUp/Sitch3DXYZ6/RouteXYZ/Attribute Function ==
  MATLAB Function : MATLAB Function  TreatAsAtomicUnit=on
  __DMLF__EDE2FCE__ : EntityDepartureFunctionCallGenerator  TimingFunctionCallF1=Before entity departure  IsInsideAFB=on
  __DMLF__GA__ : GetAttribute  AttributeName=DST_X|DST_Y|DST_Z|IME_X|IME_Y|IME_Z  AttributeMissing=Error|Error|Error|Error|Error|Error  AttributeDefaultValue=1|1|1|1|1|1  AttributeTreatAsVector=1|1|1|1|1|1  AttributeSendTiming=Before entity departure|Before entity departure|Before entity departure|Before entity departure|Before entity departure|Before entity departure  EvaluatedDefaultAttributeValue={ [];[];[];[];[];[]}  IsInsideAFB=on
      settings: OutputPortMap=o1,o2,o3,o4,o5,o6
  __DMLF__SA__ : SetAttribute  AttributeName=RT  AttributeFrom=Signal port  EvaluatedAttributeValue={ []}  IsInsideAFB=on
  IN : PMIOPort  Port=1  Side=Left
  OUT : PMIOPort  Port=2  Side=Right
  wires:
  __DMLF__EDE2FCE__/1 -> MATLAB Function/Trigger
  __DMLF__GA__/1 -> MATLAB Function/1(DST_X)
  __DMLF__GA__/2 -> MATLAB Function/2(DST_Y)
  __DMLF__GA__/3 -> MATLAB Function/3(DST_Z)
  __DMLF__GA__/4 -> MATLAB Function/4(IME_X)
  __DMLF__GA__/5 -> MATLAB Function/5(IME_Y)
  __DMLF__GA__/6 -> MATLAB Function/6(IME_Z)
  MATLAB Function/1(out_RT) -> __DMLF__SA__/1
  connections:
  __DMLF__SA__/LConn1 -- __DMLF__EDE2FCE__/RConn1
  __DMLF__GA__/RConn1 -- __DMLF__EDE2FCE__/LConn1
  IN/RConn1 -- __DMLF__GA__/LConn1
  __DMLF__SA__/RConn1 -- OUT/RConn1

== system NoC_4x4x3/LayerUp/Sitch3DXYZ7/RouteXYZ/Attribute Function ==
  MATLAB Function : MATLAB Function  TreatAsAtomicUnit=on
  __DMLF__EDE2FCE__ : EntityDepartureFunctionCallGenerator  TimingFunctionCallF1=Before entity departure  IsInsideAFB=on
  __DMLF__GA__ : GetAttribute  AttributeName=DST_X|DST_Y|DST_Z|IME_X|IME_Y|IME_Z  AttributeMissing=Error|Error|Error|Error|Error|Error  AttributeDefaultValue=1|1|1|1|1|1  AttributeTreatAsVector=1|1|1|1|1|1  AttributeSendTiming=Before entity departure|Before entity departure|Before entity departure|Before entity departure|Before entity departure|Before entity departure  EvaluatedDefaultAttributeValue={ [];[];[];[];[];[]}  IsInsideAFB=on
      settings: OutputPortMap=o1,o2,o3,o4,o5,o6
  __DMLF__SA__ : SetAttribute  AttributeName=RT  AttributeFrom=Signal port  EvaluatedAttributeValue={ []}  IsInsideAFB=on
  IN : PMIOPort  Port=1  Side=Left
  OUT : PMIOPort  Port=2  Side=Right
  wires:
  __DMLF__EDE2FCE__/1 -> MATLAB Function/Trigger
  __DMLF__GA__/1 -> MATLAB Function/1(DST_X)
  __DMLF__GA__/2 -> MATLAB Function/2(DST_Y)
  __DMLF__GA__/3 -> MATLAB Function/3(DST_Z)
  __DMLF__GA__/4 -> MATLAB Function/4(IME_X)
  __DMLF__GA__/5 -> MATLAB Function/5(IME_Y)
  __DMLF__GA__/6 -> MATLAB Function/6(IME_Z)
  MATLAB Function/1(out_RT) -> __DMLF__SA__/1
  connections:
  __DMLF__SA__/RConn1 -- OUT/RConn1
  IN/RConn1 -- __DMLF__GA__/LConn1
  __DMLF__GA__/RConn1 -- __DMLF__EDE2FCE__/LConn1
  __DMLF__SA__/LConn1 -- __DMLF__EDE2FCE__/RConn1

== system NoC_4x4x3/LayerUp/Sitch3DXYZ8/RouteXYZ/Attribute Function ==
  MATLAB Function : MATLAB Function  TreatAsAtomicUnit=on
  __DMLF__EDE2FCE__ : EntityDepartureFunctionCallGenerator  TimingFunctionCallF1=Before entity departure  IsInsideAFB=on
  __DMLF__GA__ : GetAttribute  AttributeName=DST_X|DST_Y|DST_Z|IME_X|IME_Y|IME_Z  AttributeMissing=Error|Error|Error|Error|Error|Error  AttributeDefaultValue=1|1|1|1|1|1  AttributeTreatAsVector=1|1|1|1|1|1  AttributeSendTiming=Before entity departure|Before entity departure|Before entity departure|Before entity departure|Before entity departure|Before entity departure  EvaluatedDefaultAttributeValue={ [];[];[];[];[];[]}  IsInsideAFB=on
      settings: OutputPortMap=o1,o2,o3,o4,o5,o6
  __DMLF__SA__ : SetAttribute  AttributeName=RT  AttributeFrom=Signal port  EvaluatedAttributeValue={ []}  IsInsideAFB=on
  IN : PMIOPort  Port=1  Side=Left
  OUT : PMIOPort  Port=2  Side=Right
  wires:
  __DMLF__EDE2FCE__/1 -> MATLAB Function/Trigger
  __DMLF__GA__/1 -> MATLAB Function/1(DST_X)
  __DMLF__GA__/2 -> MATLAB Function/2(DST_Y)
  __DMLF__GA__/3 -> MATLAB Function/3(DST_Z)
  __DMLF__GA__/4 -> MATLAB Function/4(IME_X)
  __DMLF__GA__/5 -> MATLAB Function/5(IME_Y)
  __DMLF__GA__/6 -> MATLAB Function/6(IME_Z)
  MATLAB Function/1(out_RT) -> __DMLF__SA__/1
  connections:
  __DMLF__SA__/RConn1 -- OUT/RConn1
  IN/RConn1 -- __DMLF__GA__/LConn1
  __DMLF__GA__/RConn1 -- __DMLF__EDE2FCE__/LConn1
  __DMLF__SA__/LConn1 -- __DMLF__EDE2FCE__/RConn1

== system NoC_4x4x3/LayerUp/Sitch3DXYZ9/RouteXYZ/Attribute Function ==
  MATLAB Function : MATLAB Function  TreatAsAtomicUnit=on
  __DMLF__EDE2FCE__ : EntityDepartureFunctionCallGenerator  TimingFunctionCallF1=Before entity departure  IsInsideAFB=on
  __DMLF__GA__ : GetAttribute  AttributeName=DST_X|DST_Y|DST_Z|IME_X|IME_Y|IME_Z  AttributeMissing=Error|Error|Error|Error|Error|Error  AttributeDefaultValue=1|1|1|1|1|1  AttributeTreatAsVector=1|1|1|1|1|1  AttributeSendTiming=Before entity departure|Before entity departure|Before entity departure|Before entity departure|Before entity departure|Before entity departure  EvaluatedDefaultAttributeValue={ [];[];[];[];[];[]}  IsInsideAFB=on
      settings: OutputPortMap=o1,o2,o3,o4,o5,o6
  __DMLF__SA__ : SetAttribute  AttributeName=RT  AttributeFrom=Signal port  EvaluatedAttributeValue={ []}  IsInsideAFB=on
  IN : PMIOPort  Port=1  Side=Left
  OUT : PMIOPort  Port=2  Side=Right
  wires:
  __DMLF__EDE2FCE__/1 -> MATLAB Function/Trigger
  __DMLF__GA__/1 -> MATLAB Function/1(DST_X)
  __DMLF__GA__/2 -> MATLAB Function/2(DST_Y)
  __DMLF__GA__/3 -> MATLAB Function/3(DST_Z)
  __DMLF__GA__/4 -> MATLAB Function/4(IME_X)
  __DMLF__GA__/5 -> MATLAB Function/5(IME_Y)
  __DMLF__GA__/6 -> MATLAB Function/6(IME_Z)
  MATLAB Function/1(out_RT) -> __DMLF__SA__/1
  connections:
  __DMLF__SA__/LConn1 -- __DMLF__EDE2FCE__/RConn1
  __DMLF__GA__/RConn1 -- __DMLF__EDE2FCE__/LConn1
  IN/RConn1 -- __DMLF__GA__/LConn1
  __DMLF__SA__/RConn1 -- OUT/RConn1

== matlab function NoC_4x4x3/Layer/Sitch3DXYZ/RouteXYZ/Attribute Function/MATLAB Function ==
  data: DST_X input; out_RT output; DST_Y input; DST_Z input; IME_X input; IME_Y input; IME_Z input
  events: trigger input FUNCTION_CALL_EVENT
function out_RT  = fcn(DST_X,DST_Y,DST_Z, IME_X, IME_Y,IME_Z)
%FCN    Access and modify attributes with MATLAB 
% 
% Input arguments must match the attribute names.
% Output arguments must be out_<AttributeName>,
% e.g., out_ServiceTime where ServiceTime is the attribute name.
% 
% The output attribute will be created if it is not present.
%

North = 1;
South = 2;
West = 3;
East = 4;
Up = 5;
Down = 6;
NI = 7;

xi =IME_X;
yi =IME_Y;
zi =IME_Z;


x = DST_X;
y = DST_Y;
z = DST_Z;

if (xi ~= x),
    if (xi < x),
        out_RT = West;
    else
        out_RT = East;
    end
elseif (yi ~= y),
    if (yi < y),
        out_RT = North;
    else
        out_RT = South;
    end
elseif (zi ~= z),
    if (zi < z),
        out_RT = Up;
    else
        out_RT = Down;
    end
else
    out_RT = NI;
end
